simulink model "Balancer"  (R2015a)
settings: Solver=ode45  StartTime=0.0  StopTime=3600*3  MaxStep=2  RelTol=1e-3
values from neighbouring files (symbols this model uses):
  BALANCE_MIN_VOLT_THRESH = 3.0    (= 3)    [Balancer_model_init.m]
  BALANCE_OFF_VOLT_TOL = 0.01    [Balancer_model_init.m]
  BALANCE_ON_VOLT_TOL = 0.1    [Balancer_model_init.m]
  CHARGE_OFF_SAFETY_MAX_VOLT = 4.15    [Balancer_model_init.m]
  CHARGE_ON_MAX_VOLT = 4.10    (= 4.1)    [Balancer_model_init.m]
  CHARGE_ON_VOLT_TOL = 0.3    [Balancer_model_init.m]
  Ibulk = 10    [Balancer_model_init.m]
  PACK_SIZE = 12    [Balancer_model_init.m]
  Q0 = (ones(1, PACK_SIZE)*Q0_nominal + Q0_variance).*PACK_NUM_PARALLEL    [Balancer_model_init.m]
  Rbalance = 0.69    [Balancer_model_init.m]
undefined symbols (not defined in the file or in its folder): BALANCE_RELAXATION_TIME
libraries: simulink x12
settings Model: Creator=abk  LastModifiedBy=abk

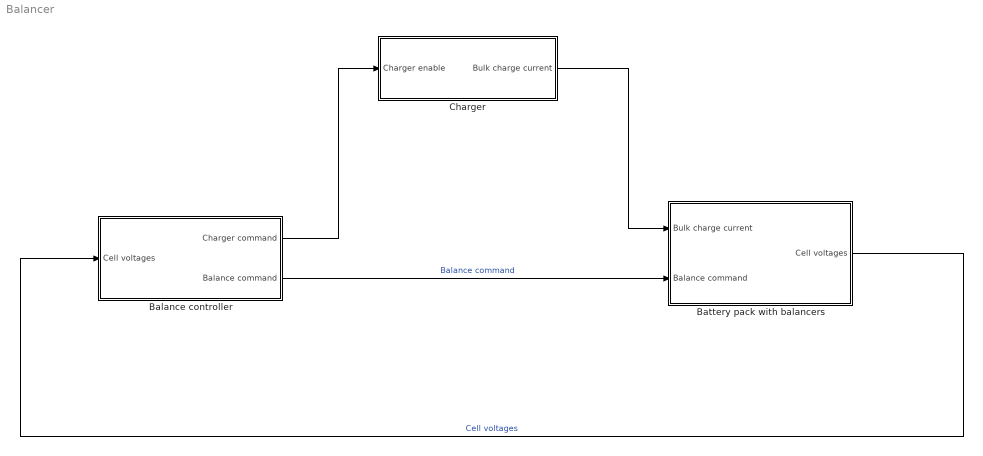
== system Balancer ==
  Balance controller : Subsystem
  Battery pack with balancers : Subsystem
  Charger : Subsystem
  wires:
  Charger/1(Bulk charge current) -> Battery pack with balancers/1(Bulk charge current)
  Balance controller/2(Balance command) -> Battery pack with balancers/2(Balance command)  "Balance command"
  Balance controller/1(Charger command) -> Charger/1(Charger enable)
  Battery pack with balancers/1(Cell voltages) -> Balance controller/1(Cell voltages)  "Cell voltages"

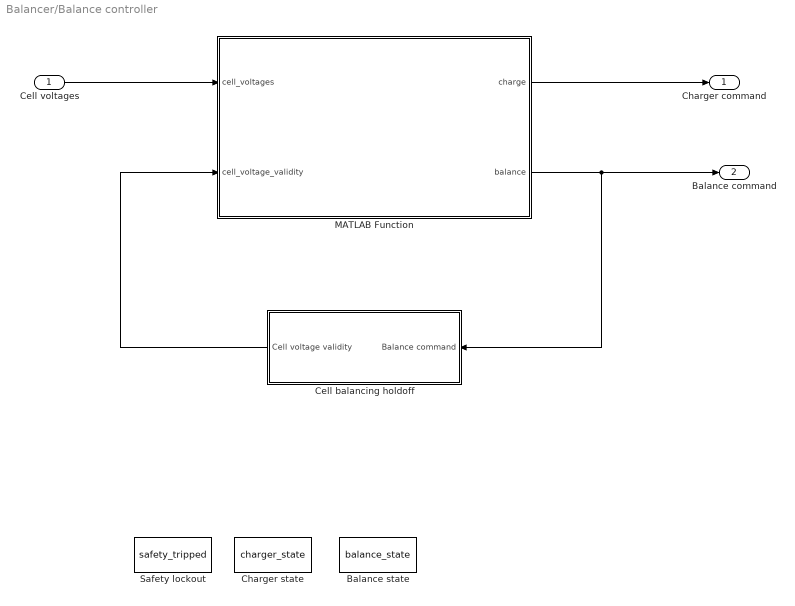
== system Balancer/Balance controller ==
  Cell voltages : Inport  PortDimensions=[1,12]
  Balance state : DataStoreMemory  DataStoreName=balance_state  InitialValue=logical(zeros(1,PACK_SIZE))  OutDataTypeStr=boolean
  Cell balancing holdoff : Subsystem
  Charger state : DataStoreMemory  DataStoreName=charger_state  OutDataTypeStr=boolean  Dimensions=1
  MATLAB Function : MATLAB Function  TreatAsAtomicUnit=on
  Safety lockout : DataStoreMemory  DataStoreName=safety_tripped  OutDataTypeStr=boolean  Dimensions=1
  Charger command : Outport
  Balance command : Outport  Port=2
  wires:
  Cell voltages/1 -> MATLAB Function/1(cell_voltages)
  MATLAB Function/1(charge) -> Charger command/1
  MATLAB Function/2(balance) -> Cell balancing holdoff/1(Balance command), Balance command/1
  Cell balancing holdoff/1(Cell voltage validity) -> MATLAB Function/2(cell_voltage_validity)

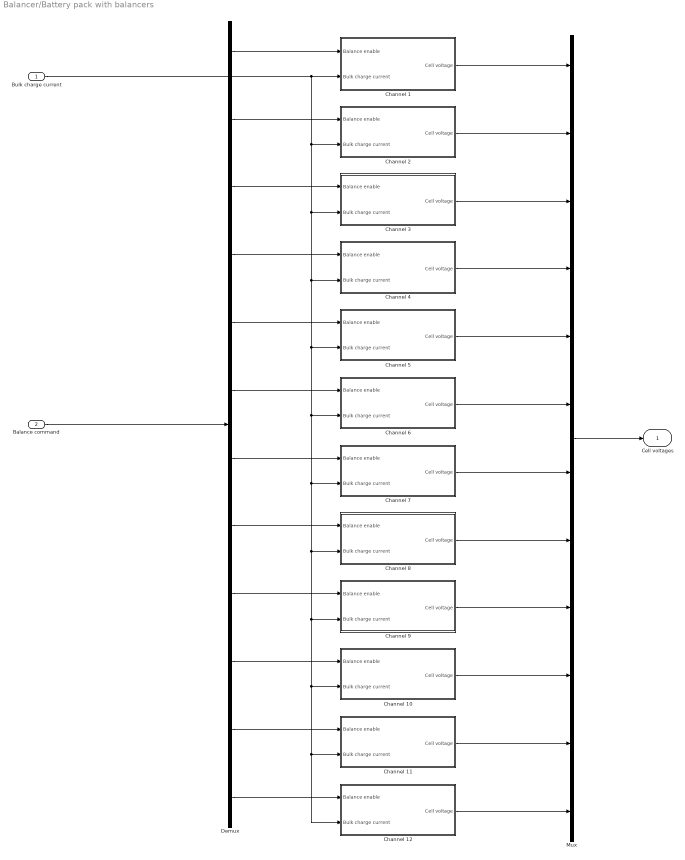
== system Balancer/Battery pack with balancers ==
  Bulk charge current : Inport
  Balance command : Inport  Port=2
  Channel 1 : Subsystem
  Channel 10 : Subsystem
  Channel 11 : Subsystem
  Channel 12 : Subsystem
  Channel 2 : Subsystem
  Channel 3 : Subsystem
  Channel 4 : Subsystem
  Channel 5 : Subsystem
  Channel 6 : Subsystem
  Channel 7 : Subsystem
  Channel 8 : Subsystem
  Channel 9 : Subsystem
  Demux : Demux  Outputs=12
  Mux : Mux  Inputs=12
  Cell voltages : Outport
  wires:
  Demux/8 -> Channel 8/1(Balance enable)
  Demux/3 -> Channel 3/1(Balance enable)
  Demux/5 -> Channel 5/1(Balance enable)
  Channel 3/1(Cell voltage) -> Mux/3
  Demux/10 -> Channel 10/1(Balance enable)
  Demux/2 -> Channel 2/1(Balance enable)
  Channel 5/1(Cell voltage) -> Mux/5
  Channel 4/1(Cell voltage) -> Mux/4
  Channel 12/1(Cell voltage) -> Mux/12
  Channel 6/1(Cell voltage) -> Mux/6
  Demux/9 -> Channel 9/1(Balance enable)
  Channel 1/1(Cell voltage) -> Mux/1
  Channel 2/1(Cell voltage) -> Mux/2
  Mux/1 -> Cell voltages/1
  Demux/12 -> Channel 12/1(Balance enable)
  Channel 11/1(Cell voltage) -> Mux/11
  Demux/11 -> Channel 11/1(Balance enable)
  Demux/4 -> Channel 4/1(Balance enable)
  Demux/6 -> Channel 6/1(Balance enable)
  Balance command/1 -> Demux/1
  Channel 7/1(Cell voltage) -> Mux/7
  Channel 9/1(Cell voltage) -> Mux/9
  Channel 10/1(Cell voltage) -> Mux/10
  Demux/7 -> Channel 7/1(Balance enable)
  Channel 8/1(Cell voltage) -> Mux/8
  Bulk charge current/1 -> Channel 12/2(Bulk charge current), Channel 11/2(Bulk charge current), Channel 10/2(Bulk charge current), Channel 9/2(Bulk charge current), Channel 8/2(Bulk charge current), Channel 7/2(Bulk charge current), Channel 6/2(Bulk charge current), Channel 5/2(Bulk charge current), Channel 4/2(Bulk charge current), Channel 3/2(Bulk charge current), Channel 2/2(Bulk charge current), Channel 1/2(Bulk charge current)
  Demux/1 -> Channel 1/1(Balance enable)

== system Balancer/Charger ==
  Charger enable : Inport
  Charge current setpoint : Constant  Value=Ibulk
  Product : Product
  Bulk charge current : Outport
  wires:
  Charger enable/1 -> Product/2
  Product/1 -> Bulk charge current/1
  Charge current setpoint/1 -> Product/1

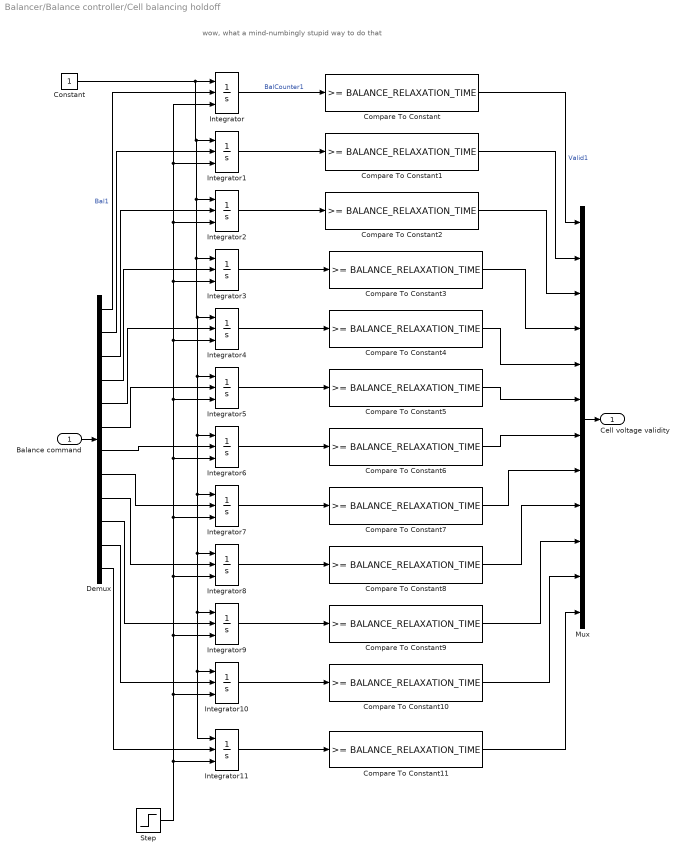
== system Balancer/Balance controller/Cell balancing holdoff ==
  note: wow, what a mind-numbingly stupid way to do that
  Balance command : Inport
  Compare To Constant{,1..11} (12 alike) : simulink/Logic and Bit Operations/Compare To Constant  relop=>=  const=BALANCE_RELAXATION_TIME  OutDataTypeStr=boolean
  Constant : Constant
  Demux : Demux  Outputs=12
  Integrator{,1..11} (12 alike) : Integrator  ExternalReset=level  InitialConditionSource=external  InitialCondition=BALANCE_RELAXATION_TIME + 1
  Mux : Mux  Inputs=12
  Step : Step  Time=5  Before=BALANCE_RELAXATION_TIME + 1  After=0  SampleTime=0
  Cell voltage validity : Outport
  wires:
  Integrator1/1 -> Compare To Constant1/1
  Integrator4/1 -> Compare To Constant4/1
  Compare To Constant10/1 -> Mux/11
  Integrator2/1 -> Compare To Constant2/1
  Integrator5/1 -> Compare To Constant5/1
  Demux/10 -> Integrator9/2
  Integrator6/1 -> Compare To Constant6/1
  Compare To Constant4/1 -> Mux/5
  Integrator8/1 -> Compare To Constant8/1
  Integrator10/1 -> Compare To Constant10/1
  Compare To Constant2/1 -> Mux/3
  Demux/2 -> Integrator1/2
  Compare To Constant3/1 -> Mux/4
  Demux/6 -> Integrator5/2
  Integrator7/1 -> Compare To Constant7/1
  Compare To Constant11/1 -> Mux/12
  Constant/1 -> Integrator1/1, Integrator2/1, Integrator3/1, Integrator4/1, Integrator5/1, Integrator6/1, Integrator7/1, Integrator8/1, Integrator9/1, Integrator11/1, Integrator10/1, Integrator/1
  Demux/4 -> Integrator3/2
  Demux/5 -> Integrator4/2
  Compare To Constant1/1 -> Mux/2
  Integrator11/1 -> Compare To Constant11/1
  Integrator3/1 -> Compare To Constant3/1
  Integrator9/1 -> Compare To Constant9/1
  Compare To Constant8/1 -> Mux/9
  Compare To Constant9/1 -> Mux/10
  Demux/3 -> Integrator2/2
  Demux/8 -> Integrator7/2
  Demux/12 -> Integrator11/2
  Mux/1 -> Cell voltage validity/1
  Compare To Constant7/1 -> Mux/8
  Balance command/1 -> Demux/1
  Demux/9 -> Integrator8/2
  Compare To Constant5/1 -> Mux/6
  Demux/7 -> Integrator6/2
  Compare To Constant/1 -> Mux/1  "Valid1"
  Demux/11 -> Integrator10/2
  Integrator/1 -> Compare To Constant/1  "BalCounter1"
  Demux/1 -> Integrator/2  "Bal1"
  Compare To Constant6/1 -> Mux/7
  Step/1 -> Integrator8/3, Integrator6/3, Integrator/3, Integrator1/3, Integrator2/3, Integrator3/3, Integrator4/3, Integrator5/3, Integrator7/3, Integrator9/3, Integrator10/3, Integrator11/3

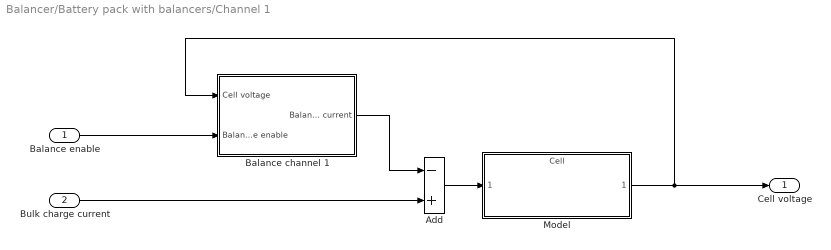
== system Balancer/Battery pack with balancers/Channel 1 ==
  Balance enable : Inport
  Bulk charge current : Inport  Port=2
  Add : Sum  Inputs=-+
  Balance channel 1 : Subsystem
  Model : ModelReference  ModelNameDialog=Cell  ParameterArgumentNames=Q0  ParameterArgumentValues=Q0(1)  SimulationMode=Normal  ModelReferenceVersion=1.4  CopyOfModelName=Cell
  Cell voltage : Outport
  wires:
  Bulk charge current/1 -> Add/2
  Balance enable/1 -> Balance channel 1/2(Balance enable)
  Balance channel 1/1(Balance current) -> Add/1
  Add/1 -> Model/1
  Model/1 -> Cell voltage/1, Balance channel 1/1(Cell voltage)

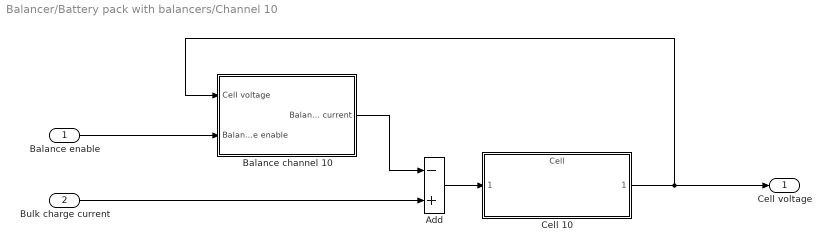
== system Balancer/Battery pack with balancers/Channel 10 ==
  Balance enable : Inport
  Bulk charge current : Inport  Port=2
  Add : Sum  Inputs=-+
  Balance channel 10 : Subsystem
  Cell 10 : ModelReference  ModelNameDialog=Cell  ParameterArgumentNames=Q0  ParameterArgumentValues=Q0(10)  SimulationMode=Normal  ModelReferenceVersion=1.4  CopyOfModelName=Cell
  Cell voltage : Outport
  wires:
  Bulk charge current/1 -> Add/2
  Balance enable/1 -> Balance channel 10/2(Balance enable)
  Balance channel 10/1(Balance current) -> Add/1
  Add/1 -> Cell 10/1
  Cell 10/1 -> Cell voltage/1, Balance channel 10/1(Cell voltage)

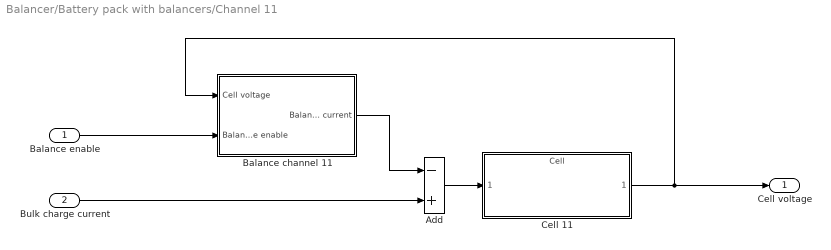
== system Balancer/Battery pack with balancers/Channel 11 ==
  Balance enable : Inport
  Bulk charge current : Inport  Port=2
  Add : Sum  Inputs=-+
  Balance channel 11 : Subsystem
  Cell 11 : ModelReference  ModelNameDialog=Cell  ParameterArgumentNames=Q0  ParameterArgumentValues=Q0(11)  SimulationMode=Normal  ModelReferenceVersion=1.4  CopyOfModelName=Cell
  Cell voltage : Outport
  wires:
  Bulk charge current/1 -> Add/2
  Balance enable/1 -> Balance channel 11/2(Balance enable)
  Balance channel 11/1(Balance current) -> Add/1
  Add/1 -> Cell 11/1
  Cell 11/1 -> Cell voltage/1, Balance channel 11/1(Cell voltage)

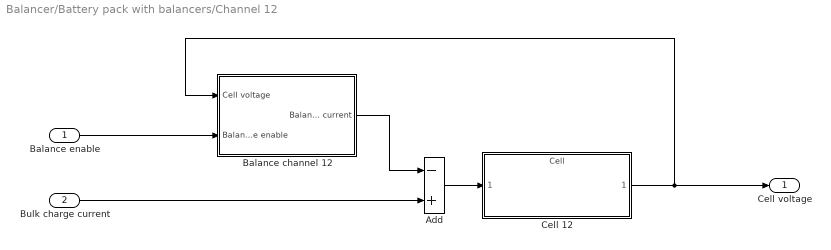
== system Balancer/Battery pack with balancers/Channel 12 ==
  Balance enable : Inport
  Bulk charge current : Inport  Port=2
  Add : Sum  Inputs=-+
  Balance channel 12 : Subsystem
  Cell 12 : ModelReference  ModelNameDialog=Cell  ParameterArgumentNames=Q0  ParameterArgumentValues=Q0(12)  SimulationMode=Normal  ModelReferenceVersion=1.4  CopyOfModelName=Cell
  Cell voltage : Outport
  wires:
  Bulk charge current/1 -> Add/2
  Balance enable/1 -> Balance channel 12/2(Balance enable)
  Balance channel 12/1(Balance current) -> Add/1
  Add/1 -> Cell 12/1
  Cell 12/1 -> Cell voltage/1, Balance channel 12/1(Cell voltage)

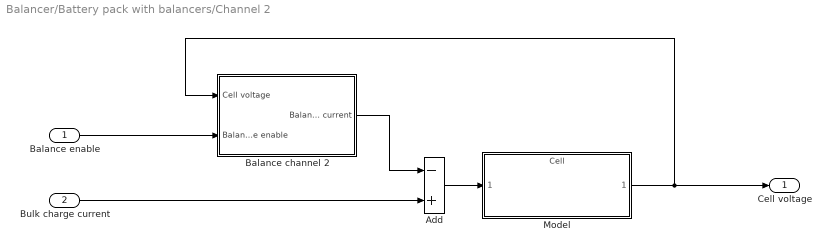
== system Balancer/Battery pack with balancers/Channel 2 ==
  Balance enable : Inport
  Bulk charge current : Inport  Port=2
  Add : Sum  Inputs=-+
  Balance channel 2 : Subsystem
  Model : ModelReference  ModelNameDialog=Cell  ParameterArgumentNames=Q0  ParameterArgumentValues=Q0(2)  SimulationMode=Normal  ModelReferenceVersion=1.4  CopyOfModelName=Cell
  Cell voltage : Outport
  wires:
  Bulk charge current/1 -> Add/2
  Balance enable/1 -> Balance channel 2/2(Balance enable)
  Balance channel 2/1(Balance current) -> Add/1
  Add/1 -> Model/1
  Model/1 -> Cell voltage/1, Balance channel 2/1(Cell voltage)

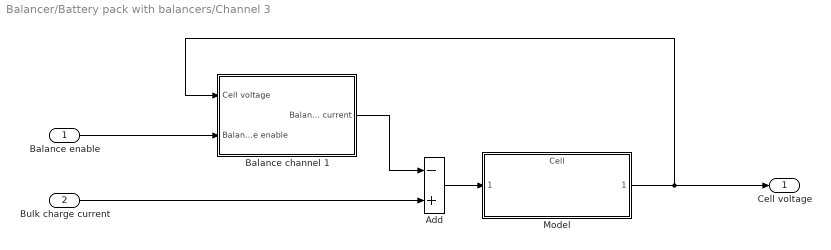
== system Balancer/Battery pack with balancers/Channel 3 ==
  Balance enable : Inport
  Bulk charge current : Inport  Port=2
  Add : Sum  Inputs=-+
  Balance channel 1 : Subsystem
  Model : ModelReference  ModelNameDialog=Cell  ParameterArgumentNames=Q0  ParameterArgumentValues=Q0(3)  SimulationMode=Normal  ModelReferenceVersion=1.4  CopyOfModelName=Cell
  Cell voltage : Outport
  wires:
  Bulk charge current/1 -> Add/2
  Balance enable/1 -> Balance channel 1/2(Balance enable)
  Balance channel 1/1(Balance current) -> Add/1
  Add/1 -> Model/1
  Model/1 -> Cell voltage/1, Balance channel 1/1(Cell voltage)

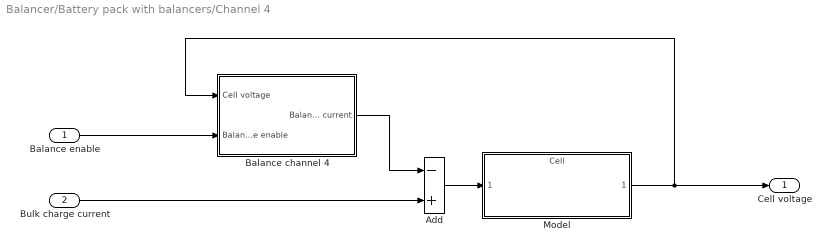
== system Balancer/Battery pack with balancers/Channel 4 ==
  Balance enable : Inport
  Bulk charge current : Inport  Port=2
  Add : Sum  Inputs=-+
  Balance channel 4 : Subsystem
  Model : ModelReference  ModelNameDialog=Cell  ParameterArgumentNames=Q0  ParameterArgumentValues=Q0(4)  SimulationMode=Normal  ModelReferenceVersion=1.4  CopyOfModelName=Cell
  Cell voltage : Outport
  wires:
  Bulk charge current/1 -> Add/2
  Balance enable/1 -> Balance channel 4/2(Balance enable)
  Balance channel 4/1(Balance current) -> Add/1
  Add/1 -> Model/1
  Model/1 -> Cell voltage/1, Balance channel 4/1(Cell voltage)

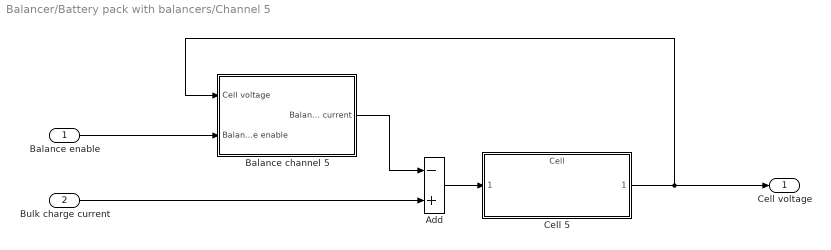
== system Balancer/Battery pack with balancers/Channel 5 ==
  Balance enable : Inport
  Bulk charge current : Inport  Port=2
  Add : Sum  Inputs=-+
  Balance channel 5 : Subsystem
  Cell 5 : ModelReference  ModelNameDialog=Cell  ParameterArgumentNames=Q0  ParameterArgumentValues=Q0(5)  SimulationMode=Normal  ModelReferenceVersion=1.4  CopyOfModelName=Cell
  Cell voltage : Outport
  wires:
  Bulk charge current/1 -> Add/2
  Balance enable/1 -> Balance channel 5/2(Balance enable)
  Balance channel 5/1(Balance current) -> Add/1
  Add/1 -> Cell 5/1
  Cell 5/1 -> Cell voltage/1, Balance channel 5/1(Cell voltage)

== system Balancer/Battery pack with balancers/Channel 6 ==
  Balance enable : Inport
  Bulk charge current : Inport  Port=2
  Add : Sum  Inputs=-+
  Balance channel 6 : Subsystem
  Cell 6 : ModelReference  ModelNameDialog=Cell  ParameterArgumentNames=Q0  ParameterArgumentValues=Q0(6)  SimulationMode=Normal  ModelReferenceVersion=1.4  CopyOfModelName=Cell
  Cell voltage : Outport
  wires:
  Bulk charge current/1 -> Add/2
  Balance enable/1 -> Balance channel 6/2(Balance enable)
  Balance channel 6/1(Balance current) -> Add/1
  Add/1 -> Cell 6/1
  Cell 6/1 -> Cell voltage/1, Balance channel 6/1(Cell voltage)

== system Balancer/Battery pack with balancers/Channel 7 ==
  Balance enable : Inport
  Bulk charge current : Inport  Port=2
  Add : Sum  Inputs=-+
  Balance channel 7 : Subsystem
  Cell 7 : ModelReference  ModelNameDialog=Cell  ParameterArgumentNames=Q0  ParameterArgumentValues=Q0(7)  SimulationMode=Normal  ModelReferenceVersion=1.4  CopyOfModelName=Cell
  Cell voltage : Outport
  wires:
  Bulk charge current/1 -> Add/2
  Balance enable/1 -> Balance channel 7/2(Balance enable)
  Balance channel 7/1(Balance current) -> Add/1
  Add/1 -> Cell 7/1
  Cell 7/1 -> Cell voltage/1, Balance channel 7/1(Cell voltage)

== system Balancer/Battery pack with balancers/Channel 8 ==
  Balance enable : Inport
  Bulk charge current : Inport  Port=2
  Add : Sum  Inputs=-+
  Balance channel 8 : Subsystem
  Cell 8 : ModelReference  ModelNameDialog=Cell  ParameterArgumentNames=Q0  ParameterArgumentValues=Q0(8)  SimulationMode=Normal  ModelReferenceVersion=1.4  CopyOfModelName=Cell
  Cell voltage : Outport
  wires:
  Bulk charge current/1 -> Add/2
  Balance enable/1 -> Balance channel 8/2(Balance enable)
  Balance channel 8/1(Balance current) -> Add/1
  Add/1 -> Cell 8/1
  Cell 8/1 -> Cell voltage/1, Balance channel 8/1(Cell voltage)

== system Balancer/Battery pack with balancers/Channel 9 ==
  Balance enable : Inport
  Bulk charge current : Inport  Port=2
  Add : Sum  Inputs=-+
  Balance channel 9 : Subsystem
  Cell 9 : ModelReference  ModelNameDialog=Cell  ParameterArgumentNames=Q0  ParameterArgumentValues=Q0(9)  SimulationMode=Normal  ModelReferenceVersion=1.4  CopyOfModelName=Cell
  Cell voltage : Outport
  wires:
  Bulk charge current/1 -> Add/2
  Balance enable/1 -> Balance channel 9/2(Balance enable)
  Balance channel 9/1(Balance current) -> Add/1
  Add/1 -> Cell 9/1
  Cell 9/1 -> Cell voltage/1, Balance channel 9/1(Cell voltage)

== system Balancer/Battery pack with balancers/Channel 1/Balance channel 1 ==
  Cell voltage : Inport
  Balance enable : Inport  Port=2
  Balance enable/disable : Product
  Memory : Memory
  "V -> I" : Gain  Gain=1/Rbalance
  Balance current : Outport
  wires:
  "V -> I"/1 -> Balance enable/disable/1
  Balance enable/disable/1 -> Balance current/1
  Cell voltage/1 -> Memory/1
  Balance enable/1 -> Balance enable/disable/2
  Memory/1 -> "V -> I"/1

== system Balancer/Battery pack with balancers/Channel 10/Balance channel 10 ==
  Cell voltage : Inport
  Balance enable : Inport  Port=2
  Balance enable/disable : Product
  Memory : Memory
  "V -> I" : Gain  Gain=1/Rbalance
  Balance current : Outport
  wires:
  "V -> I"/1 -> Balance enable/disable/1
  Balance enable/disable/1 -> Balance current/1
  Cell voltage/1 -> Memory/1
  Balance enable/1 -> Balance enable/disable/2
  Memory/1 -> "V -> I"/1

== system Balancer/Battery pack with balancers/Channel 11/Balance channel 11 ==
  Cell voltage : Inport
  Balance enable : Inport  Port=2
  Balance enable/disable : Product
  Memory : Memory
  "V -> I" : Gain  Gain=1/Rbalance
  Balance current : Outport
  wires:
  "V -> I"/1 -> Balance enable/disable/1
  Balance enable/disable/1 -> Balance current/1
  Cell voltage/1 -> Memory/1
  Balance enable/1 -> Balance enable/disable/2
  Memory/1 -> "V -> I"/1

== system Balancer/Battery pack with balancers/Channel 12/Balance channel 12 ==
  Cell voltage : Inport
  Balance enable : Inport  Port=2
  Balance enable/disable : Product
  Memory : Memory
  "V -> I" : Gain  Gain=1/Rbalance
  Balance current : Outport
  wires:
  "V -> I"/1 -> Balance enable/disable/1
  Balance enable/disable/1 -> Balance current/1
  Cell voltage/1 -> Memory/1
  Balance enable/1 -> Balance enable/disable/2
  Memory/1 -> "V -> I"/1

== system Balancer/Battery pack with balancers/Channel 2/Balance channel 2 ==
  Cell voltage : Inport
  Balance enable : Inport  Port=2
  Balance enable/disable : Product
  Memory : Memory
  "V -> I" : Gain  Gain=1/Rbalance
  Balance current : Outport
  wires:
  "V -> I"/1 -> Balance enable/disable/1
  Balance enable/disable/1 -> Balance current/1
  Cell voltage/1 -> Memory/1
  Balance enable/1 -> Balance enable/disable/2
  Memory/1 -> "V -> I"/1

== system Balancer/Battery pack with balancers/Channel 3/Balance channel 1 ==
  Cell voltage : Inport
  Balance enable : Inport  Port=2
  Balance enable/disable : Product
  Memory : Memory
  "V -> I" : Gain  Gain=1/Rbalance
  Balance current : Outport
  wires:
  "V -> I"/1 -> Balance enable/disable/1
  Balance enable/disable/1 -> Balance current/1
  Cell voltage/1 -> Memory/1
  Balance enable/1 -> Balance enable/disable/2
  Memory/1 -> "V -> I"/1

== system Balancer/Battery pack with balancers/Channel 4/Balance channel 4 ==
  Cell voltage : Inport
  Balance enable : Inport  Port=2
  Balance enable/disable : Product
  Memory : Memory
  "V -> I" : Gain  Gain=1/Rbalance
  Balance current : Outport
  wires:
  "V -> I"/1 -> Balance enable/disable/1
  Balance enable/disable/1 -> Balance current/1
  Cell voltage/1 -> Memory/1
  Balance enable/1 -> Balance enable/disable/2
  Memory/1 -> "V -> I"/1

== system Balancer/Battery pack with balancers/Channel 5/Balance channel 5 ==
  Cell voltage : Inport
  Balance enable : Inport  Port=2
  Balance enable/disable : Product
  Memory : Memory
  "V -> I" : Gain  Gain=1/Rbalance
  Balance current : Outport
  wires:
  "V -> I"/1 -> Balance enable/disable/1
  Balance enable/disable/1 -> Balance current/1
  Cell voltage/1 -> Memory/1
  Balance enable/1 -> Balance enable/disable/2
  Memory/1 -> "V -> I"/1

== system Balancer/Battery pack with balancers/Channel 6/Balance channel 6 ==
  Cell voltage : Inport
  Balance enable : Inport  Port=2
  Balance enable/disable : Product
  Memory : Memory
  "V -> I" : Gain  Gain=1/Rbalance
  Balance current : Outport
  wires:
  "V -> I"/1 -> Balance enable/disable/1
  Balance enable/disable/1 -> Balance current/1
  Cell voltage/1 -> Memory/1
  Balance enable/1 -> Balance enable/disable/2
  Memory/1 -> "V -> I"/1

== system Balancer/Battery pack with balancers/Channel 7/Balance channel 7 ==
  Cell voltage : Inport
  Balance enable : Inport  Port=2
  Balance enable/disable : Product
  Memory : Memory
  "V -> I" : Gain  Gain=1/Rbalance
  Balance current : Outport
  wires:
  "V -> I"/1 -> Balance enable/disable/1
  Balance enable/disable/1 -> Balance current/1
  Cell voltage/1 -> Memory/1
  Balance enable/1 -> Balance enable/disable/2
  Memory/1 -> "V -> I"/1

== system Balancer/Battery pack with balancers/Channel 8/Balance channel 8 ==
  Cell voltage : Inport
  Balance enable : Inport  Port=2
  Balance enable/disable : Product
  Memory : Memory
  "V -> I" : Gain  Gain=1/Rbalance
  Balance current : Outport
  wires:
  "V -> I"/1 -> Balance enable/disable/1
  Balance enable/disable/1 -> Balance current/1
  Cell voltage/1 -> Memory/1
  Balance enable/1 -> Balance enable/disable/2
  Memory/1 -> "V -> I"/1

== system Balancer/Battery pack with balancers/Channel 9/Balance channel 9 ==
  Cell voltage : Inport
  Balance enable : Inport  Port=2
  Balance enable/disable : Product
  Memory : Memory
  "V -> I" : Gain  Gain=1/Rbalance
  Balance current : Outport
  wires:
  "V -> I"/1 -> Balance enable/disable/1
  Balance enable/disable/1 -> Balance current/1
  Cell voltage/1 -> Memory/1
  Balance enable/1 -> Balance enable/disable/2
  Memory/1 -> "V -> I"/1

== matlab function Balancer/Balance controller/MATLAB Function ==
  data: cell_voltages input size=[1 12]; charge output; balance output size=[1, PACK_SIZE]; CHARGE_OFF_SAFETY_MAX_VOLT parameter; PACK_SIZE parameter; CHARGE_ON_MAX_VOLT parameter; CHARGE_ON_VOLT_TOL parameter; charger_state data_store_memory; balance_state data_store_memory; safety_tripped data_store_memory; BALANCE_MIN_VOLT_THRESH parameter; BALANCE_ON_VOLT_TOL parameter; BALANCE_OFF_VOLT_TOL parameter; cell_voltage_validity input size=[1,12]
function [charge, balance] = fcn(cell_voltages, CHARGE_OFF_SAFETY_MAX_VOLT, PACK_SIZE, CHARGE_ON_MAX_VOLT, CHARGE_ON_VOLT_TOL, BALANCE_MIN_VOLT_THRESH, BALANCE_ON_VOLT_TOL, BALANCE_OFF_VOLT_TOL, cell_voltage_validity)
%#codegen

global charger_state balance_state safety_tripped;

cell_voltages = cell_voltages';

%% Charger control
% Simple hysteresis to enable/disable bulk charging
if( ~charger_state )		
	% Charger currently off.
	if( all( cell_voltages < CHARGE_ON_MAX_VOLT - CHARGE_ON_VOLT_TOL ) )
		charge = true;
	else
		charge = false;
	end
else
	% Charger currently on.
	if( all(cell_voltages < CHARGE_ON_MAX_VOLT) )
		charge = true;
	else
		charge = false;
	end
end

% Disable charging permanently if safety check fails.
if( any( cell_voltages > CHARGE_OFF_SAFETY_MAX_VOLT ) )
	charge = false;
	safety_tripped = true;
end

if( safety_tripped )
	charge = false;
end

%% Balance control

if( ~any(cell_voltage_validity' & ~balance_state) )
	% No cells are eligible to be target voltages
	% No balancing for you
	balance = logical( zeros(1, PACK_SIZE) );
else
	% Only consider cells not currently balancing as min cells
	% AND cells that have not been balanced in BALANCE_RELAXATION_TIME seconds
	minCellVolt		= min( cell_voltages(~balance_state & cell_voltage_validity') );	

	% Determine which cells to turn on
	not_balancing	= ~balance_state;
	to_enable		=	cell_voltages > BALANCE_MIN_VOLT_THRESH &	...			% Cell voltage above minimum threshold
						not_balancing &								...			% Not currently balancing
						(cell_voltages - minCellVolt) > BALANCE_ON_VOLT_TOL;	% Above the minimum cell by the threshold

	% Determine which cells to turn off
	to_disable		=	cell_voltages < BALANCE_MIN_VOLT_THRESH |	...			% Turn off if below minimum voltage threshold
						(cell_voltages - minCellVolt) < BALANCE_OFF_VOLT_TOL;	% or if cell becomes close enough to min cell
	to_disable		=	to_disable & balance_state;								% Only apply these conditions to currently balancing cells

	balance			= ((balance_state | to_enable) & ~to_disable)';

	% balance = logical( zeros(1, PACK_SIZE) );		% Disable balancing
end

charger_state	= charge;
balance_state	= balance';

end
